simulink model "q20a"  (R2016a)
settings: Solver=VariableStepAuto  StartTime=0.0  StopTime=10.0  RelTol=1e-3
settings Model: Creator=Satya  LastModifiedBy=Satya

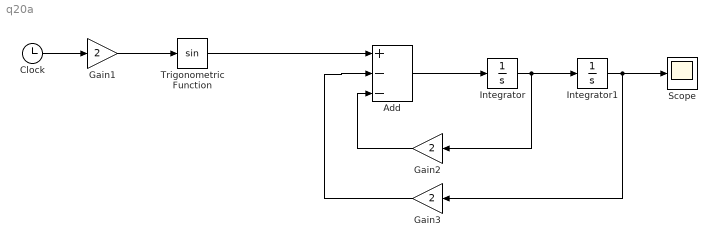
== system q20a ==
  Add : Sum  Inputs=+--
  Clock : Clock
  Gain1 : Gain  Gain=2
  Gain2 : Gain  Gain=2
  Gain3 : Gain  Gain=2
  Integrator : Integrator  InitialCondition=-3
  Integrator1 : Integrator  InitialCondition=2
  Scope : Scope
  Trigonometric Function : Trigonometry
  wires:
  Integrator/1 -> Gain2/1, Integrator1/1
  Integrator1/1 -> Gain3/1, Scope/1
  Add/1 -> Integrator/1
  Trigonometric Function/1 -> Add/1
  Gain2/1 -> Add/3
  Gain3/1 -> Add/2
  Clock/1 -> Gain1/1
  Gain1/1 -> Trigonometric Function/1
